simulink model "gm_parallel_prediction_and_cost_function_6phase"  (R2022a)
settings: Solver=FixedStepDiscrete  StartTime=0.0  StopTime=10.0  RelTol=1e-3
undefined symbols (not defined in the file or in its folder): f_c, L_d, L_q, L_x, L_y, p, psi_pm, R_ph
libraries: hdlmdlgenlib x2
(part 2 of 8)

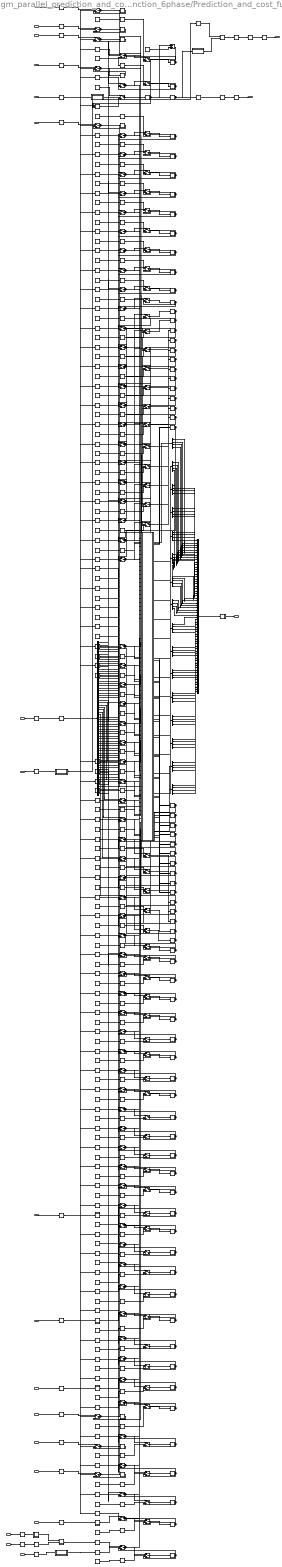
== system gm_parallel_prediction_and_cost_function_6phase/Prediction_and_cost_function ==
  Lq_AXI : Inport  OutDataTypeStr=single  PortDimensions=1  SampleTime=1e-08
  Ld_AXI : Inport  Port=2  OutDataTypeStr=single  PortDimensions=1  SampleTime=1e-08
  SampleTime_div_Ld_AXI : Inport  Port=3  OutDataTypeStr=single  PortDimensions=1  SampleTime=1e-08
  SampleTime_div_Lq_AXI : Inport  Port=4  OutDataTypeStr=single  PortDimensions=1  SampleTime=1e-08
  SampleTime_div_Lx_AXI : Inport  Port=5  OutDataTypeStr=single  PortDimensions=1  SampleTime=1e-08
  SampleTime_div_Ly_AXI : Inport  Port=6  OutDataTypeStr=single  PortDimensions=1  SampleTime=1e-08
  id_k_1 : Inport  Port=7  OutDataTypeStr=fixdt(1, 18, 11)  PortDimensions=1  SampleTime=1e-08
  iq_k_1 : Inport  Port=8  OutDataTypeStr=fixdt(1, 18, 11)  PortDimensions=1  SampleTime=1e-08
  ix_k_1 : Inport  Port=9  OutDataTypeStr=fixdt(1, 18, 11)  PortDimensions=1  SampleTime=1e-08
  iy_k_1 : Inport  Port=10  OutDataTypeStr=fixdt(1, 18, 11)  PortDimensions=1  SampleTime=1e-08
  Rs_AXI : Inport  Port=11  OutDataTypeStr=single  PortDimensions=1  SampleTime=1e-08
  omega_m_measured : Inport  Port=12  OutDataTypeStr=fixdt(1, 24, 11)  PortDimensions=1  SampleTime=1e-08
  pole_pairs_AXI : Inport  Port=13  OutDataTypeStr=single  PortDimensions=1  SampleTime=1e-08
  psiPM_AXI : Inport  Port=14  OutDataTypeStr=single  PortDimensions=1  SampleTime=1e-08
  valid_in : Inport  Port=15  OutDataTypeStr=boolean  PortDimensions=1  SampleTime=1e-08
  Reset : Inport  Port=16  OutDataTypeStr=boolean  PortDimensions=1  SampleTime=1e-08
  valid_in_ADC : Inport  Port=17  OutDataTypeStr=boolean  PortDimensions=1  SampleTime=1e-08
  dqxy_phase_voltage_per_switching_state : Inport  Port=18  OutDataTypeStr=fixdt(1, 24, 11)  PortDimensions=[64]  SampleTime=1e-08
  Compare To Constant : Subsystem  mask(Compare To Constant){relop=<=, const=double(4), OutDataTypeStr=boolean, ZeroCross=on}
      mask prompts: relop "Simulink:masks:Operator_MP"; const "Simulink:masks:ConstantValue_MP"; OutDataTypeStr "Simulink:masks:OutputDataType_MP"; ZeroCross "Simulink:masks:EnableZerocrossingDetection_MP"
      mask help: Simulink:masks:CompareToConstant_MD
      mask init:
      | OutDataTypeStr = 'boolean';
      | ZeroCross = 'on';
      | blkName = 'parallel_prediction_and_cost_function_6phase/Prediction_and_cost_function/Compare\nTo Constant';
      | const = double(4);
      | const_str = '4';
      | const_val = double(4);
      | relop = '<=';
      | setValue = 'boolean';
      | str = '<= 4';
      mask TypeOptions relop: == | ~= | < | <= | >= | >
      mask TypeOptions OutDataTypeStr: Simulink:masks:uint8 | Simulink:masks:boolean
      mask Callback ZeroCross: sl('zeroCrossEnable', gcbh);
      mask Display: disp(str)
  Data Type Conversion1 : Subsystem
      mask Display: disp('NFP\nconv');
  Data Type Conversion10 : Subsystem
      mask Display: disp('NFP\nconv');
  Data Type Conversion18 : Subsystem
      mask Display: disp('NFP\nconv');
  Data Type Conversion4 : Subsystem
      mask Display: disp('NFP\nconv');
  Data Type Conversion7 : Subsystem
      mask Display: disp('NFP\nconv');
  Data Type Conversion8 : Subsystem
      mask Display: disp('NFP\nconv');
  Data Type Conversion9 : Subsystem
      mask Display: disp('NFP\nconv');
  Delay{4..32,34..37,51,57,59..60,76..135} (97 alike) : Delay  DelayLength=double(1)  InitialCondition=0  SampleTime=1e-08
  Delay100_enbsw : Switch  Criteria=u2 ~= 0  Threshold=double(0)  OutDataTypeStr=single  SampleTime=1e-08  SaturateOnIntegerOverflow=off  InputSameDT=off
  Delay101_enbsw : Switch  Criteria=u2 ~= 0  Threshold=double(0)  OutDataTypeStr=single  SampleTime=1e-08  SaturateOnIntegerOverflow=off  InputSameDT=off
  Delay102_enbsw : Switch  Criteria=u2 ~= 0  Threshold=double(0)  OutDataTypeStr=single  SampleTime=1e-08  SaturateOnIntegerOverflow=off  InputSameDT=off
  Delay103_enbsw : Switch  Criteria=u2 ~= 0  Threshold=double(0)  OutDataTypeStr=single  SampleTime=1e-08  SaturateOnIntegerOverflow=off  InputSameDT=off
  Delay104_enbsw : Switch  Criteria=u2 ~= 0  Threshold=double(0)  OutDataTypeStr=single  SampleTime=1e-08  SaturateOnIntegerOverflow=off  InputSameDT=off
  Delay105_enbsw : Switch  Criteria=u2 ~= 0  Threshold=double(0)  OutDataTypeStr=single  SampleTime=1e-08  SaturateOnIntegerOverflow=off  InputSameDT=off
  Delay106_enbsw : Switch  Criteria=u2 ~= 0  Threshold=double(0)  OutDataTypeStr=single  SampleTime=1e-08  SaturateOnIntegerOverflow=off  InputSameDT=off
  Delay107_enbsw : Switch  Criteria=u2 ~= 0  Threshold=double(0)  OutDataTypeStr=single  SampleTime=1e-08  SaturateOnIntegerOverflow=off  InputSameDT=off
  Delay108_enbsw : Switch  Criteria=u2 ~= 0  Threshold=double(0)  OutDataTypeStr=single  SampleTime=1e-08  SaturateOnIntegerOverflow=off  InputSameDT=off
  Delay109_enbsw : Switch  Criteria=u2 ~= 0  Threshold=double(0)  OutDataTypeStr=single  SampleTime=1e-08  SaturateOnIntegerOverflow=off  InputSameDT=off
  Delay110_enbsw : Switch  Criteria=u2 ~= 0  Threshold=double(0)  OutDataTypeStr=single  SampleTime=1e-08  SaturateOnIntegerOverflow=off  InputSameDT=off
  Delay111_enbsw : Switch  Criteria=u2 ~= 0  Threshold=double(0)  OutDataTypeStr=single  SampleTime=1e-08  SaturateOnIntegerOverflow=off  InputSameDT=off
  Delay112_enbsw : Switch  Criteria=u2 ~= 0  Threshold=double(0)  OutDataTypeStr=single  SampleTime=1e-08  SaturateOnIntegerOverflow=off  InputSameDT=off
  Delay113_enbsw : Switch  Criteria=u2 ~= 0  Threshold=double(0)  OutDataTypeStr=single  SampleTime=1e-08  SaturateOnIntegerOverflow=off  InputSameDT=off
  Delay114_enbsw : Switch  Criteria=u2 ~= 0  Threshold=double(0)  OutDataTypeStr=single  SampleTime=1e-08  SaturateOnIntegerOverflow=off  InputSameDT=off
  Delay115_enbsw : Switch  Criteria=u2 ~= 0  Threshold=double(0)  OutDataTypeStr=single  SampleTime=1e-08  SaturateOnIntegerOverflow=off  InputSameDT=off
  Delay116_enbsw : Switch  Criteria=u2 ~= 0  Threshold=double(0)  OutDataTypeStr=single  SampleTime=1e-08  SaturateOnIntegerOverflow=off  InputSameDT=off
  Delay117_enbsw : Switch  Criteria=u2 ~= 0  Threshold=double(0)  OutDataTypeStr=single  SampleTime=1e-08  SaturateOnIntegerOverflow=off  InputSameDT=off
  Delay118_enbsw : Switch  Criteria=u2 ~= 0  Threshold=double(0)  OutDataTypeStr=single  SampleTime=1e-08  SaturateOnIntegerOverflow=off  InputSameDT=off
  Delay119_enbsw : Switch  Criteria=u2 ~= 0  Threshold=double(0)  OutDataTypeStr=single  SampleTime=1e-08  SaturateOnIntegerOverflow=off  InputSameDT=off
  Delay11_enbsw : Switch  Criteria=u2 ~= 0  Threshold=double(0)  OutDataTypeStr=single  SampleTime=1e-08  SaturateOnIntegerOverflow=off  InputSameDT=off
  Delay120_enbsw : Switch  Criteria=u2 ~= 0  Threshold=double(0)  OutDataTypeStr=single  SampleTime=1e-08  SaturateOnIntegerOverflow=off  InputSameDT=off
  Delay121_enbsw : Switch  Criteria=u2 ~= 0  Threshold=double(0)  OutDataTypeStr=single  SampleTime=1e-08  SaturateOnIntegerOverflow=off  InputSameDT=off
  Delay122_enbsw : Switch  Criteria=u2 ~= 0  Threshold=double(0)  OutDataTypeStr=single  SampleTime=1e-08  SaturateOnIntegerOverflow=off  InputSameDT=off
  Delay123_enbsw : Switch  Criteria=u2 ~= 0  Threshold=double(0)  OutDataTypeStr=single  SampleTime=1e-08  SaturateOnIntegerOverflow=off  InputSameDT=off
  Delay124_enbsw : Switch  Criteria=u2 ~= 0  Threshold=double(0)  OutDataTypeStr=single  SampleTime=1e-08  SaturateOnIntegerOverflow=off  InputSameDT=off
  Delay125_enbsw : Switch  Criteria=u2 ~= 0  Threshold=double(0)  OutDataTypeStr=single  SampleTime=1e-08  SaturateOnIntegerOverflow=off  InputSameDT=off
  Delay126_enbsw : Switch  Criteria=u2 ~= 0  Threshold=double(0)  OutDataTypeStr=single  SampleTime=1e-08  SaturateOnIntegerOverflow=off  InputSameDT=off
  Delay127_enbsw : Switch  Criteria=u2 ~= 0  Threshold=double(0)  OutDataTypeStr=single  SampleTime=1e-08  SaturateOnIntegerOverflow=off  InputSameDT=off
  Delay128_enbsw : Switch  Criteria=u2 ~= 0  Threshold=double(0)  OutDataTypeStr=single  SampleTime=1e-08  SaturateOnIntegerOverflow=off  InputSameDT=off
  Delay129_enbsw : Switch  Criteria=u2 ~= 0  Threshold=double(0)  OutDataTypeStr=single  SampleTime=1e-08  SaturateOnIntegerOverflow=off  InputSameDT=off
  Delay130_enbsw : Switch  Criteria=u2 ~= 0  Threshold=double(0)  OutDataTypeStr=single  SampleTime=1e-08  SaturateOnIntegerOverflow=off  InputSameDT=off
  Delay131_enbsw : Switch  Criteria=u2 ~= 0  Threshold=double(0)  OutDataTypeStr=single  SampleTime=1e-08  SaturateOnIntegerOverflow=off  InputSameDT=off
  Delay132_enbsw : Switch  Criteria=u2 ~= 0  Threshold=double(0)  OutDataTypeStr=single  SampleTime=1e-08  SaturateOnIntegerOverflow=off  InputSameDT=off
  Delay133_enbsw : Switch  Criteria=u2 ~= 0  Threshold=double(0)  OutDataTypeStr=single  SampleTime=1e-08  SaturateOnIntegerOverflow=off  InputSameDT=off
  Delay134_enbsw : Switch  Criteria=u2 ~= 0  Threshold=double(0)  OutDataTypeStr=single  SampleTime=1e-08  SaturateOnIntegerOverflow=off  InputSameDT=off
  Delay135_enbsw : Switch  Criteria=u2 ~= 0  Threshold=double(0)  OutDataTypeStr=single  SampleTime=1e-08  SaturateOnIntegerOverflow=off  InputSameDT=off
  Delay13_enbsw : Switch  Criteria=u2 ~= 0  Threshold=double(0)  OutDataTypeStr=single  SampleTime=1e-08  SaturateOnIntegerOverflow=off  InputSameDT=off
  Delay14_enbsw : Switch  Criteria=u2 ~= 0  Threshold=double(0)  OutDataTypeStr=single  SampleTime=1e-08  SaturateOnIntegerOverflow=off  InputSameDT=off
  Delay15_enbsw : Switch  Criteria=u2 ~= 0  Threshold=double(0)  OutDataTypeStr=single  SampleTime=1e-08  SaturateOnIntegerOverflow=off  InputSameDT=off
  Delay16_enbsw : Switch  Criteria=u2 ~= 0  Threshold=double(0)  OutDataTypeStr=single  SampleTime=1e-08  SaturateOnIntegerOverflow=off  InputSameDT=off
  Delay4_enbsw : Switch  Criteria=u2 ~= 0  Threshold=double(0)  OutDataTypeStr=single  SampleTime=1e-08  SaturateOnIntegerOverflow=off  InputSameDT=off
  Delay58 : Delay  DelayLength=double(3)  InitialCondition=0  SampleTime=1e-08
  Delay5_enbsw : Switch  Criteria=u2 ~= 0  Threshold=double(0)  OutDataTypeStr=single  SampleTime=1e-08  SaturateOnIntegerOverflow=off  InputSameDT=off
  Delay6_enbsw : Switch  Criteria=u2 ~= 0  Threshold=double(0)  OutDataTypeStr=single  SampleTime=1e-08  SaturateOnIntegerOverflow=off  InputSameDT=off
  Delay76_enbsw : Switch  Criteria=u2 ~= 0  Threshold=double(0)  OutDataTypeStr=single  SampleTime=1e-08  SaturateOnIntegerOverflow=off  InputSameDT=off
  Delay77_enbsw : Switch  Criteria=u2 ~= 0  Threshold=double(0)  OutDataTypeStr=single  SampleTime=1e-08  SaturateOnIntegerOverflow=off  InputSameDT=off
  Delay78_enbsw : Switch  Criteria=u2 ~= 0  Threshold=double(0)  OutDataTypeStr=single  SampleTime=1e-08  SaturateOnIntegerOverflow=off  InputSameDT=off
  Delay79_enbsw : Switch  Criteria=u2 ~= 0  Threshold=double(0)  OutDataTypeStr=single  SampleTime=1e-08  SaturateOnIntegerOverflow=off  InputSameDT=off
  Delay7_enbsw : Switch  Criteria=u2 ~= 0  Threshold=double(0)  OutDataTypeStr=single  SampleTime=1e-08  SaturateOnIntegerOverflow=off  InputSameDT=off
  Delay80_enbsw : Switch  Criteria=u2 ~= 0  Threshold=double(0)  OutDataTypeStr=single  SampleTime=1e-08  SaturateOnIntegerOverflow=off  InputSameDT=off
  Delay81_enbsw : Switch  Criteria=u2 ~= 0  Threshold=double(0)  OutDataTypeStr=single  SampleTime=1e-08  SaturateOnIntegerOverflow=off  InputSameDT=off
  Delay82_enbsw : Switch  Criteria=u2 ~= 0  Threshold=double(0)  OutDataTypeStr=single  SampleTime=1e-08  SaturateOnIntegerOverflow=off  InputSameDT=off
  Delay83_enbsw : Switch  Criteria=u2 ~= 0  Threshold=double(0)  OutDataTypeStr=single  SampleTime=1e-08  SaturateOnIntegerOverflow=off  InputSameDT=off
  Delay84_enbsw : Switch  Criteria=u2 ~= 0  Threshold=double(0)  OutDataTypeStr=single  SampleTime=1e-08  SaturateOnIntegerOverflow=off  InputSameDT=off
  Delay85_enbsw : Switch  Criteria=u2 ~= 0  Threshold=double(0)  OutDataTypeStr=single  SampleTime=1e-08  SaturateOnIntegerOverflow=off  InputSameDT=off
  Delay86_enbsw : Switch  Criteria=u2 ~= 0  Threshold=double(0)  OutDataTypeStr=single  SampleTime=1e-08  SaturateOnIntegerOverflow=off  InputSameDT=off
  Delay87_enbsw : Switch  Criteria=u2 ~= 0  Threshold=double(0)  OutDataTypeStr=single  SampleTime=1e-08  SaturateOnIntegerOverflow=off  InputSameDT=off
  Delay88_enbsw : Switch  Criteria=u2 ~= 0  Threshold=double(0)  OutDataTypeStr=single  SampleTime=1e-08  SaturateOnIntegerOverflow=off  InputSameDT=off
  Delay89_enbsw : Switch  Criteria=u2 ~= 0  Threshold=double(0)  OutDataTypeStr=single  SampleTime=1e-08  SaturateOnIntegerOverflow=off  InputSameDT=off
  Delay90_enbsw : Switch  Criteria=u2 ~= 0  Threshold=double(0)  OutDataTypeStr=single  SampleTime=1e-08  SaturateOnIntegerOverflow=off  InputSameDT=off
  Delay91_enbsw : Switch  Criteria=u2 ~= 0  Threshold=double(0)  OutDataTypeStr=single  SampleTime=1e-08  SaturateOnIntegerOverflow=off  InputSameDT=off
  Delay92_enbsw : Switch  Criteria=u2 ~= 0  Threshold=double(0)  OutDataTypeStr=single  SampleTime=1e-08  SaturateOnIntegerOverflow=off  InputSameDT=off
  Delay93_enbsw : Switch  Criteria=u2 ~= 0  Threshold=double(0)  OutDataTypeStr=single  SampleTime=1e-08  SaturateOnIntegerOverflow=off  InputSameDT=off
  Delay94_enbsw : Switch  Criteria=u2 ~= 0  Threshold=double(0)  OutDataTypeStr=single  SampleTime=1e-08  SaturateOnIntegerOverflow=off  InputSameDT=off
  Delay95_enbsw : Switch  Criteria=u2 ~= 0  Threshold=double(0)  OutDataTypeStr=single  SampleTime=1e-08  SaturateOnIntegerOverflow=off  InputSameDT=off
  Delay96_enbsw : Switch  Criteria=u2 ~= 0  Threshold=double(0)  OutDataTypeStr=single  SampleTime=1e-08  SaturateOnIntegerOverflow=off  InputSameDT=off
  Delay97_enbsw : Switch  Criteria=u2 ~= 0  Threshold=double(0)  OutDataTypeStr=single  SampleTime=1e-08  SaturateOnIntegerOverflow=off  InputSameDT=off
  Delay98_enbsw : Switch  Criteria=u2 ~= 0  Threshold=double(0)  OutDataTypeStr=single  SampleTime=1e-08  SaturateOnIntegerOverflow=off  InputSameDT=off
  Delay99_enbsw : Switch  Criteria=u2 ~= 0  Threshold=double(0)  OutDataTypeStr=single  SampleTime=1e-08  SaturateOnIntegerOverflow=off  InputSameDT=off
  Detect Rise Positive : Subsystem  mask(Detect Rise Positive){vinit=double(0), InputProcessing=Elements as channels (sample based), OutDataTypeStr=boolean}
      mask prompts: vinit "Simulink:masks:InitialCondition_MP"; InputProcessing "Simulink:masks:InputProcessing_MP"; OutDataTypeStr "Simulink:masks:OutputDataType_MP"
      mask help: Simulink:masks:DetectRisePositive_MD
      mask init:
      | InputProcessing = 'Elements as channels (sample based)';
      | OutDataTypeStr = 'boolean';
      | vinit = double(0);
      mask TypeOptions InputProcessing: Simulink:masks:ColumnsAsChannelsFrameBased | Simulink:masks:ElementsAsChannelsSampleBased
      mask TypeOptions OutDataTypeStr: Simulink:masks:uint8 | Simulink:masks:boolean
      mask Display: fprintf('U > 0\n&  NOT\nU/z > 0')
  Detect Rise Positive1 : Subsystem  mask(Detect Rise Positive){vinit=double(0), InputProcessing=Elements as channels (sample based), OutDataTypeStr=boolean}
      mask prompts: vinit "Simulink:masks:InitialCondition_MP"; InputProcessing "Simulink:masks:InputProcessing_MP"; OutDataTypeStr "Simulink:masks:OutputDataType_MP"
      mask help: Simulink:masks:DetectRisePositive_MD
      mask init:
      | InputProcessing = 'Elements as channels (sample based)';
      | OutDataTypeStr = 'boolean';
      | vinit = double(0);
      mask TypeOptions InputProcessing: Simulink:masks:ColumnsAsChannelsFrameBased | Simulink:masks:ElementsAsChannelsSampleBased
      mask TypeOptions OutDataTypeStr: Simulink:masks:uint8 | Simulink:masks:boolean
      mask Display: fprintf('U > 0\n&  NOT\nU/z > 0')
  Detect Rise Positive2 : Subsystem  mask(Detect Rise Positive){vinit=double(0), InputProcessing=Elements as channels (sample based), OutDataTypeStr=boolean}
      mask prompts: vinit "Simulink:masks:InitialCondition_MP"; InputProcessing "Simulink:masks:InputProcessing_MP"; OutDataTypeStr "Simulink:masks:OutputDataType_MP"
      mask help: Simulink:masks:DetectRisePositive_MD
      mask init:
      | InputProcessing = 'Elements as channels (sample based)';
      | OutDataTypeStr = 'boolean';
      | vinit = double(0);
      mask TypeOptions InputProcessing: Simulink:masks:ColumnsAsChannelsFrameBased | Simulink:masks:ElementsAsChannelsSampleBased
      mask TypeOptions OutDataTypeStr: Simulink:masks:uint8 | Simulink:masks:boolean
      mask Display: fprintf('U > 0\n&  NOT\nU/z > 0')
  HDL Counter : Delay  DelayLength=double(1)  InitialCondition=0  SampleTime=1e-08
  HDL Counter_out1 : hdlmdlgenlib/Buffer
      settings: SourceProductBaseCode=SL
  Logical Operator : Logic  AllPortsSameDT=off  OutDataTypeStr=boolean  SampleTime=1e-08
  Product : Subsystem
      mask Display: disp('NFP\nmul');
  Product_outbuff : hdlmdlgenlib/Buffer
      settings: SourceProductBaseCode=SL
  Subsystem : Subsystem
  Switch_on{4..13,15..21,31..90} (77 alike) : Switch  Threshold=double(1)  OutDataTypeStr=single  RndMeth=Simplest  SampleTime=1e-08  SaturateOnIntegerOverflow=off  InputSameDT=off
  adder : Sum  AccumDataTypeStr=int32  OutDataTypeStr=int32  SampleTime=1e-08
  const : Constant  Value=0  VectorParams1D=off  OutDataTypeStr=int32  SampleTime=1e-08
  delayMatch : Delay  DelayLength=double(36)  InitialCondition=0  SampleTime=1e-08
  delayMatch1 : Delay  DelayLength=double(36)  InitialCondition=0  SampleTime=1e-08
  delayMatch{2..130,133..140} (137 alike) : Delay  DelayLength=double(6)  InitialCondition=0  SampleTime=1e-08
  delayMatch131 : Delay  DelayLength=double(12)  InitialCondition=0  SampleTime=1e-08
  delayMatch132 : Delay  DelayLength=double(12)  InitialCondition=0  SampleTime=1e-08
  delayMatch141 : Delay  DelayLength=double(11)  InitialCondition=0  SampleTime=1e-08
  delayMatch142 : Delay  DelayLength=double(11)  InitialCondition=0  SampleTime=1e-08
  mux : Mux  Inputs=64
  stateControl{,1..68} (69 alike) : Constant  OutDataTypeStr=boolean  SampleTime=1e-08
  step_value : Constant  VectorParams1D=off  OutDataTypeStr=int32  SampleTime=1e-08
  switchEnable : MultiPortSwitch  DataPortOrder=Zero-based contiguous  Inputs=2  DiagnosticForDefault=None  zeroidx=on  OutDataTypeStr=int32  SampleTime=1e-08  SaturateOnIntegerOverflow=off  InputSameDT=off
  switchReset : Switch  Criteria=u2 ~= 0  Threshold=double(0)  OutDataTypeStr=int32  SampleTime=1e-08  SaturateOnIntegerOverflow=off  InputSameDT=off
  t : Demux  Outputs=64
  t{1..16} (16 alike) : Demux
  done : Outport  SampleTime=1e-08
  Index : Outport  Port=2  SampleTime=1e-08
  Prediction : Outport  Port=3  SampleTime=1e-08
  wires:
  Lq_AXI/1 -> Delay34/1
  Ld_AXI/1 -> Delay36/1
  SampleTime_div_Ld_AXI/1 -> Delay23/1
  SampleTime_div_Lq_AXI/1 -> Delay24/1
  SampleTime_div_Lx_AXI/1 -> Delay25/1
  SampleTime_div_Ly_AXI/1 -> Delay26/1
  id_k_1/1 -> Delay27/1
  iq_k_1/1 -> Delay28/1
  ix_k_1/1 -> Delay29/1
  iy_k_1/1 -> Delay30/1
  Rs_AXI/1 -> Delay31/1
  omega_m_measured/1 -> Delay51/1
  pole_pairs_AXI/1 -> Delay35/1
  psiPM_AXI/1 -> Delay37/1
  valid_in/1 -> Delay21/1
  Reset/1 -> Delay57/1
  valid_in_ADC/1 -> Delay60/1
  dqxy_phase_voltage_per_switching_state/1 -> Delay32/1
  Compare To Constant/1(y) -> Logical Operator/2
  Delay21/1 -> Detect Rise Positive/1(U)
  Delay22/1 -> Logical Operator/1
  Delay23/1 -> Switch_on21/1
  Delay24/1 -> Switch_on20/1
  Delay25/1 -> Switch_on19/1
  Delay26/1 -> Switch_on18/1
  Delay27/1 -> Data Type Conversion7/1(In1)
  Delay28/1 -> Data Type Conversion8/1(In1)
  Delay29/1 -> Data Type Conversion9/1(In1)
  Delay30/1 -> Data Type Conversion10/1(In1)
  Delay31/1 -> Switch_on12/1
  Delay32/1 -> Data Type Conversion1/1(In1)
  Delay34/1 -> Switch_on10/1
  delayMatch130/1 -> Product/2(In2)
  Delay36/1 -> Switch_on9/1
  Delay37/1 -> Switch_on8/1
  Delay51/1 -> Data Type Conversion4/1(In1)
  Delay57/1 -> Detect Rise Positive1/1(U)
  delayMatch141/1 -> done/1
  delayMatch142/1 -> Index/1
  Delay60/1 -> Detect Rise Positive2/1(U)
  delayMatch3/1 -> Switch_on90/2
  Detect Rise Positive1/1(Y) -> switchReset/2
  delayMatch132/1 -> Switch_on11/2
  HDL Counter_out1/1 -> Delay59/1, Compare To Constant/1(u)
  Logical Operator/1 -> Delay58/1
  mux/1 -> Data Type Conversion18/1(In1)
  Product_outbuff/1 -> Switch_on11/1
  Subsystem/1(Prediction_1) -> t1/1
  Subsystem/2(Prediction_2) -> t2/1
  Subsystem/3(Prediction_3) -> t3/1
  Subsystem/4(Prediction_4) -> t4/1
  Subsystem/5(Prediction_5) -> t5/1
  Subsystem/6(Prediction_6) -> t6/1
  Subsystem/7(Prediction_7) -> t7/1
  Subsystem/8(Prediction_8) -> t8/1
  Subsystem/9(Prediction_9) -> t9/1
  Subsystem/10(Prediction_10) -> t10/1
  Subsystem/11(Prediction_11) -> t11/1
  Subsystem/12(Prediction_12) -> t12/1
  Subsystem/13(Prediction_13) -> t13/1
  Subsystem/14(Prediction_14) -> t14/1
  Subsystem/15(Prediction_15) -> t15/1
  Subsystem/16(Prediction_16) -> t16/1
  Switch_on10/1 -> Subsystem/71(Lq15), Delay10/1
  Switch_on12/1 -> Subsystem/69(Rs15), Delay12/1
  Switch_on18/1 -> Subsystem/64(SampleTime_div_Ly15), Delay17/1
  Switch_on19/1 -> Subsystem/63(SampleTime_div_Lx15), Delay18/1
  Switch_on20/1 -> Subsystem/62(SampleTime_div_Lq15), Delay19/1
  Switch_on21/1 -> Subsystem/61(SampleTime_div_Ld15), Delay20/1
  Switch_on8/1 -> Subsystem/73(psiPM15), Delay8/1
  Switch_on9/1 -> Subsystem/72(Ld15), Delay9/1
  HDL Counter/1 -> HDL Counter_out1/1, switchEnable/2, adder/1
  const/1 -> switchReset/1
  step_value/1 -> adder/2
  t/1 -> Switch_on90/1
  t/2 -> Switch_on89/1
  t/3 -> Switch_on88/1
  t/4 -> Switch_on87/1
  t/5 -> Switch_on86/1
  t/6 -> Switch_on85/1
  t/7 -> Switch_on84/1
  t/8 -> Switch_on83/1
  t/9 -> Switch_on82/1
  t/10 -> Switch_on81/1
  t/11 -> Switch_on80/1
  t/12 -> Switch_on79/1
  t/13 -> Switch_on78/1
  t/14 -> Switch_on77/1
  t/15 -> Switch_on76/1
  t/16 -> Switch_on75/1
  t/17 -> Switch_on74/1
  t/18 -> Switch_on73/1
  t/19 -> Switch_on72/1
  t/20 -> Switch_on71/1
  t/21 -> Switch_on70/1
  t/22 -> Switch_on69/1
  t/23 -> Switch_on68/1
  t/24 -> Switch_on67/1
  t/25 -> Switch_on66/1
  t/26 -> Switch_on65/1
  t/27 -> Switch_on64/1
  t/28 -> Switch_on63/1
  t/29 -> Switch_on62/1
  t/30 -> Switch_on61/1
  t/31 -> Switch_on60/1
  t/32 -> Switch_on59/1
  t/33 -> Switch_on58/1
  t/34 -> Switch_on57/1
  t/35 -> Switch_on56/1
  t/36 -> Switch_on55/1
  t/37 -> Switch_on54/1
  t/38 -> Switch_on53/1
  t/39 -> Switch_on52/1
  t/40 -> Switch_on51/1
  t/41 -> Switch_on50/1
  t/42 -> Switch_on49/1
  t/43 -> Switch_on48/1
  t/44 -> Switch_on47/1
  t/45 -> Switch_on46/1
  t/46 -> Switch_on45/1
  t/47 -> Switch_on44/1
  t/48 -> Switch_on43/1
  t/49 -> Switch_on42/1
  t/50 -> Switch_on41/1
  t/51 -> Switch_on40/1
  t/52 -> Switch_on39/1
  t/53 -> Switch_on38/1
  t/54 -> Switch_on37/1
  t/55 -> Switch_on36/1
  t/56 -> Switch_on35/1
  t/57 -> Switch_on34/1
  t/58 -> Switch_on33/1
  t/59 -> Switch_on32/1
  t/60 -> Switch_on31/1
  t/61 -> Switch_on7/1
  t/62 -> Switch_on6/1
  t/63 -> Switch_on5/1
  t/64 -> Switch_on4/1
  t1/1 -> mux/1
  t1/2 -> mux/2
  t1/3 -> mux/3
  t1/4 -> mux/4
  t2/1 -> mux/5
  t2/2 -> mux/6
  t2/3 -> mux/7
  t2/4 -> mux/8
  t3/1 -> mux/9
  t3/2 -> mux/10
  t3/3 -> mux/11
  t3/4 -> mux/12
  t4/1 -> mux/13
  t4/2 -> mux/14
  t4/3 -> mux/15
  t4/4 -> mux/16
  t5/1 -> mux/17
  t5/2 -> mux/18
  t5/3 -> mux/19
  t5/4 -> mux/20
  t6/1 -> mux/21
  t6/2 -> mux/22
  t6/3 -> mux/23
  t6/4 -> mux/24
  t7/1 -> mux/25
  t7/2 -> mux/26
  t7/3 -> mux/27
  t7/4 -> mux/28
  t8/1 -> mux/29
  t8/2 -> mux/30
  t8/3 -> mux/31
  t8/4 -> mux/32
  t9/1 -> mux/33
  t9/2 -> mux/34
  t9/3 -> mux/35
  t9/4 -> mux/36
  t10/1 -> mux/37
  t10/2 -> mux/38
  t10/3 -> mux/39
  t10/4 -> mux/40
  t11/1 -> mux/41
  t11/2 -> mux/42
  t11/3 -> mux/43
  t11/4 -> mux/44
  t12/1 -> mux/45
  t12/2 -> mux/46
  t12/3 -> mux/47
  t12/4 -> mux/48
  t13/1 -> mux/49
  t13/2 -> mux/50
  t13/3 -> mux/51
  t13/4 -> mux/52
  t14/1 -> mux/53
  t14/2 -> mux/54
  t14/3 -> mux/55
  t14/4 -> mux/56
  t15/1 -> mux/57
  t15/2 -> mux/58
  t15/3 -> mux/59
  t15/4 -> mux/60
  t16/1 -> mux/61
  t16/2 -> mux/62
  t16/3 -> mux/63
  t16/4 -> mux/64
  Delay58/1 -> delayMatch/1
  Delay59/1 -> delayMatch1/1
  Data Type Conversion1/1(Out1) -> t/1
  Data Type Conversion10/1(Out1) -> Switch_on13/1
  Data Type Conversion18/1(Out1) -> Prediction/1
  Data Type Conversion4/1(Out1) -> Product/1(In1)
  Data Type Conversion7/1(Out1) -> Switch_on17/1
  Data Type Conversion8/1(Out1) -> Switch_on16/1
  Data Type Conversion9/1(Out1) -> Switch_on15/1
  Product/1(Out1) -> Product_outbuff/1
  delayMatch2/1 -> Delay135_enbsw/2
  delayMatch4/1 -> Delay134_enbsw/2
  delayMatch6/1 -> Delay133_enbsw/2
  delayMatch8/1 -> Delay132_enbsw/2
  delayMatch10/1 -> Delay131_enbsw/2
  delayMatch12/1 -> Delay130_enbsw/2
  delayMatch14/1 -> Delay129_enbsw/2
  delayMatch16/1 -> Delay128_enbsw/2
  delayMatch18/1 -> Delay127_enbsw/2
  delayMatch20/1 -> Delay126_enbsw/2
  delayMatch22/1 -> Delay125_enbsw/2
  delayMatch24/1 -> Delay124_enbsw/2
  delayMatch26/1 -> Delay123_enbsw/2
  delayMatch28/1 -> Delay122_enbsw/2
  delayMatch30/1 -> Delay121_enbsw/2
  delayMatch32/1 -> Delay120_enbsw/2
  delayMatch34/1 -> Delay119_enbsw/2
  delayMatch36/1 -> Delay118_enbsw/2
  delayMatch38/1 -> Delay117_enbsw/2
  delayMatch40/1 -> Delay116_enbsw/2
  delayMatch42/1 -> Delay115_enbsw/2
  delayMatch44/1 -> Delay114_enbsw/2
  delayMatch46/1 -> Delay113_enbsw/2
  delayMatch48/1 -> Delay112_enbsw/2
  delayMatch50/1 -> Delay111_enbsw/2
  delayMatch52/1 -> Delay110_enbsw/2
  delayMatch54/1 -> Delay109_enbsw/2
  delayMatch56/1 -> Delay108_enbsw/2
  delayMatch58/1 -> Delay107_enbsw/2
  delayMatch60/1 -> Delay106_enbsw/2
  delayMatch62/1 -> Delay105_enbsw/2
  delayMatch64/1 -> Delay104_enbsw/2
  delayMatch66/1 -> Delay103_enbsw/2
  delayMatch68/1 -> Delay102_enbsw/2
  delayMatch70/1 -> Delay101_enbsw/2
  delayMatch72/1 -> Delay100_enbsw/2
  delayMatch74/1 -> Delay99_enbsw/2
  delayMatch76/1 -> Delay98_enbsw/2
  delayMatch78/1 -> Delay97_enbsw/2
  delayMatch80/1 -> Delay96_enbsw/2
  delayMatch82/1 -> Delay95_enbsw/2
  delayMatch84/1 -> Delay94_enbsw/2
  delayMatch86/1 -> Delay93_enbsw/2
  delayMatch88/1 -> Delay92_enbsw/2
  delayMatch90/1 -> Delay91_enbsw/2
  delayMatch92/1 -> Delay90_enbsw/2
  delayMatch94/1 -> Delay89_enbsw/2
  delayMatch96/1 -> Delay88_enbsw/2
  delayMatch98/1 -> Delay87_enbsw/2
  delayMatch100/1 -> Delay86_enbsw/2
  delayMatch102/1 -> Delay85_enbsw/2
  delayMatch104/1 -> Delay84_enbsw/2
  delayMatch106/1 -> Delay83_enbsw/2
  delayMatch108/1 -> Delay82_enbsw/2
  delayMatch110/1 -> Delay81_enbsw/2
  delayMatch112/1 -> Delay80_enbsw/2
  delayMatch114/1 -> Delay79_enbsw/2
  delayMatch116/1 -> Delay78_enbsw/2
  delayMatch118/1 -> Delay77_enbsw/2
  delayMatch120/1 -> Delay76_enbsw/2
  delayMatch122/1 -> Delay16_enbsw/2
  delayMatch124/1 -> Delay15_enbsw/2
  delayMatch126/1 -> Delay14_enbsw/2
  delayMatch128/1 -> Delay13_enbsw/2
  delayMatch131/1 -> Delay11_enbsw/2
  delayMatch133/1 -> Delay7_enbsw/2
  delayMatch135/1 -> Delay6_enbsw/2
  delayMatch137/1 -> Delay5_enbsw/2
  delayMatch139/1 -> Delay4_enbsw/2
  stateControl/1 -> delayMatch2/1
  delayMatch5/1 -> Switch_on89/2
  stateControl1/1 -> delayMatch4/1
  delayMatch7/1 -> Switch_on88/2
  stateControl2/1 -> delayMatch6/1
  delayMatch9/1 -> Switch_on87/2
  stateControl3/1 -> delayMatch8/1
  delayMatch11/1 -> Switch_on86/2
  stateControl4/1 -> delayMatch10/1
  delayMatch13/1 -> Switch_on85/2
  stateControl5/1 -> delayMatch12/1
  delayMatch15/1 -> Switch_on84/2
  stateControl6/1 -> delayMatch14/1
  delayMatch17/1 -> Switch_on83/2
  stateControl7/1 -> delayMatch16/1
  delayMatch19/1 -> Switch_on82/2
  stateControl8/1 -> delayMatch18/1
  delayMatch21/1 -> Switch_on81/2
  stateControl9/1 -> delayMatch20/1
  delayMatch23/1 -> Switch_on80/2
  stateControl10/1 -> delayMatch22/1
  delayMatch25/1 -> Switch_on79/2
  stateControl11/1 -> delayMatch24/1
  delayMatch27/1 -> Switch_on78/2
  stateControl12/1 -> delayMatch26/1
  delayMatch29/1 -> Switch_on77/2
  stateControl13/1 -> delayMatch28/1
  delayMatch31/1 -> Switch_on76/2
  stateControl14/1 -> delayMatch30/1
  delayMatch33/1 -> Switch_on75/2
  stateControl15/1 -> delayMatch32/1
  delayMatch35/1 -> Switch_on74/2
  stateControl16/1 -> delayMatch34/1
  delayMatch37/1 -> Switch_on73/2
  stateControl17/1 -> delayMatch36/1
  delayMatch39/1 -> Switch_on72/2
  stateControl18/1 -> delayMatch38/1
  delayMatch41/1 -> Switch_on71/2
  stateControl19/1 -> delayMatch40/1
  delayMatch43/1 -> Switch_on70/2
  stateControl20/1 -> delayMatch42/1
  delayMatch45/1 -> Switch_on69/2
  stateControl21/1 -> delayMatch44/1
  delayMatch47/1 -> Switch_on68/2
  stateControl22/1 -> delayMatch46/1
  delayMatch49/1 -> Switch_on67/2
  stateControl23/1 -> delayMatch48/1
  delayMatch51/1 -> Switch_on66/2
  stateControl24/1 -> delayMatch50/1
  delayMatch53/1 -> Switch_on65/2
  stateControl25/1 -> delayMatch52/1
  delayMatch55/1 -> Switch_on64/2
  stateControl26/1 -> delayMatch54/1
  delayMatch57/1 -> Switch_on63/2
  stateControl27/1 -> delayMatch56/1
  delayMatch59/1 -> Switch_on62/2
  stateControl28/1 -> delayMatch58/1
  delayMatch61/1 -> Switch_on61/2
  stateControl29/1 -> delayMatch60/1
  delayMatch63/1 -> Switch_on60/2
  stateControl30/1 -> delayMatch62/1
  delayMatch65/1 -> Switch_on59/2
  stateControl31/1 -> delayMatch64/1
  delayMatch67/1 -> Switch_on58/2
  stateControl32/1 -> delayMatch66/1
  delayMatch69/1 -> Switch_on57/2
  stateControl33/1 -> delayMatch68/1
  delayMatch71/1 -> Switch_on56/2
  stateControl34/1 -> delayMatch70/1
  delayMatch73/1 -> Switch_on55/2
  stateControl35/1 -> delayMatch72/1
  delayMatch75/1 -> Switch_on54/2
  stateControl36/1 -> delayMatch74/1
  delayMatch77/1 -> Switch_on53/2
  stateControl37/1 -> delayMatch76/1
  delayMatch79/1 -> Switch_on52/2
  stateControl38/1 -> delayMatch78/1
  delayMatch81/1 -> Switch_on51/2
  stateControl39/1 -> delayMatch80/1
  delayMatch83/1 -> Switch_on50/2
  stateControl40/1 -> delayMatch82/1
  delayMatch85/1 -> Switch_on49/2
  stateControl41/1 -> delayMatch84/1
  delayMatch87/1 -> Switch_on48/2
  stateControl42/1 -> delayMatch86/1
  delayMatch89/1 -> Switch_on47/2
  stateControl43/1 -> delayMatch88/1
  delayMatch91/1 -> Switch_on46/2
  stateControl44/1 -> delayMatch90/1
  delayMatch93/1 -> Switch_on45/2
  stateControl45/1 -> delayMatch92/1
  delayMatch95/1 -> Switch_on44/2
  stateControl46/1 -> delayMatch94/1
  delayMatch97/1 -> Switch_on43/2
  stateControl47/1 -> delayMatch96/1
  delayMatch99/1 -> Switch_on42/2
  stateControl48/1 -> delayMatch98/1
  delayMatch101/1 -> Switch_on41/2
  stateControl49/1 -> delayMatch100/1
  delayMatch103/1 -> Switch_on40/2
  stateControl50/1 -> delayMatch102/1
  delayMatch105/1 -> Switch_on39/2
  stateControl51/1 -> delayMatch104/1
  delayMatch107/1 -> Switch_on38/2
  stateControl52/1 -> delayMatch106/1
  delayMatch109/1 -> Switch_on37/2
  stateControl53/1 -> delayMatch108/1
  delayMatch111/1 -> Switch_on36/2
  stateControl54/1 -> delayMatch110/1
  delayMatch113/1 -> Switch_on35/2
  stateControl55/1 -> delayMatch112/1
  delayMatch115/1 -> Switch_on34/2
  stateControl56/1 -> delayMatch114/1
  delayMatch117/1 -> Switch_on33/2
  stateControl57/1 -> delayMatch116/1
  delayMatch119/1 -> Switch_on32/2
  stateControl58/1 -> delayMatch118/1
  delayMatch121/1 -> Switch_on31/2
  stateControl59/1 -> delayMatch120/1
  delayMatch123/1 -> Switch_on17/2
  stateControl60/1 -> delayMatch122/1
  delayMatch125/1 -> Switch_on16/2
  stateControl61/1 -> delayMatch124/1
  delayMatch127/1 -> Switch_on15/2
  stateControl62/1 -> delayMatch126/1
  delayMatch129/1 -> Switch_on13/2
  stateControl63/1 -> delayMatch128/1
  delayMatch134/1 -> Switch_on7/2
  Delay35/1 -> delayMatch130/1
  stateControl64/1 -> delayMatch131/1
  Detect Rise Positive2/1(Y) -> delayMatch132/1
  stateControl65/1 -> delayMatch133/1
  delayMatch136/1 -> Switch_on6/2
  stateControl66/1 -> delayMatch135/1
  delayMatch138/1 -> Switch_on5/2
  stateControl67/1 -> delayMatch137/1
  delayMatch140/1 -> Switch_on4/2
  stateControl68/1 -> delayMatch139/1
  Detect Rise Positive/1(Y) -> delayMatch140/1, delayMatch138/1, delayMatch136/1, delayMatch134/1, delayMatch129/1, delayMatch127/1, delayMatch125/1, delayMatch123/1, delayMatch121/1, delayMatch119/1, delayMatch117/1, delayMatch115/1, delayMatch113/1, delayMatch111/1, delayMatch109/1, delayMatch107/1, delayMatch105/1, delayMatch103/1, delayMatch101/1, delayMatch99/1, delayMatch97/1, delayMatch95/1, delayMatch93/1, delayMatch91/1, delayMatch89/1, delayMatch87/1, delayMatch85/1, delayMatch83/1, delayMatch81/1, delayMatch79/1, delayMatch77/1, delayMatch75/1, delayMatch73/1, delayMatch71/1, delayMatch69/1, delayMatch67/1, delayMatch65/1, delayMatch63/1, delayMatch61/1, delayMatch59/1, delayMatch57/1, delayMatch55/1, delayMatch53/1, delayMatch51/1, delayMatch49/1, delayMatch47/1, delayMatch45/1, delayMatch43/1, delayMatch41/1, delayMatch39/1, delayMatch37/1, delayMatch35/1, delayMatch33/1, delayMatch31/1, delayMatch29/1, delayMatch27/1, delayMatch25/1, delayMatch23/1, delayMatch21/1, delayMatch19/1, delayMatch17/1, delayMatch15/1, delayMatch13/1, delayMatch11/1, delayMatch9/1, delayMatch7/1, delayMatch5/1, delayMatch3/1, Delay22/1, switchEnable/1, Switch_on21/2, Switch_on20/2, Switch_on19/2, Switch_on18/2, Switch_on12/2, Switch_on10/2, Switch_on9/2, Switch_on8/2
  delayMatch/1 -> delayMatch141/1
  delayMatch1/1 -> delayMatch142/1
  Switch_on90/1 -> Subsystem/1(d_phase_voltage_per_switching_state), Delay135_enbsw/1
  Switch_on89/1 -> Subsystem/2(q_phase_voltage_per_switching_state), Delay134_enbsw/1
  Switch_on88/1 -> Subsystem/3(x_phase_voltage_per_switching_state), Delay133_enbsw/1
  Switch_on87/1 -> Subsystem/4(y_phase_voltage_per_switching_state), Delay132_enbsw/1
  Switch_on86/1 -> Subsystem/5(d_phase_voltage_per_switching_state1), Delay131_enbsw/1
  Switch_on85/1 -> Subsystem/6(q_phase_voltage_per_switching_state1), Delay130_enbsw/1
  Switch_on84/1 -> Subsystem/7(x_phase_voltage_per_switching_state1), Delay129_enbsw/1
  Switch_on83/1 -> Subsystem/8(y_phase_voltage_per_switching_state1), Delay128_enbsw/1
  Switch_on82/1 -> Subsystem/9(d_phase_voltage_per_switching_state2), Delay127_enbsw/1
  Switch_on81/1 -> Subsystem/10(q_phase_voltage_per_switching_state2), Delay126_enbsw/1
  Switch_on80/1 -> Subsystem/11(x_phase_voltage_per_switching_state2), Delay125_enbsw/1
  Switch_on79/1 -> Subsystem/12(y_phase_voltage_per_switching_state2), Delay124_enbsw/1
  Switch_on78/1 -> Subsystem/13(d_phase_voltage_per_switching_state3), Delay123_enbsw/1
  Switch_on77/1 -> Subsystem/14(q_phase_voltage_per_switching_state3), Delay122_enbsw/1
  Switch_on76/1 -> Subsystem/15(x_phase_voltage_per_switching_state3), Delay121_enbsw/1
  Switch_on75/1 -> Subsystem/16(y_phase_voltage_per_switching_state3), Delay120_enbsw/1
  Switch_on74/1 -> Subsystem/17(d_phase_voltage_per_switching_state4), Delay119_enbsw/1
  Switch_on73/1 -> Subsystem/18(q_phase_voltage_per_switching_state4), Delay118_enbsw/1
  Switch_on72/1 -> Subsystem/19(x_phase_voltage_per_switching_state4), Delay117_enbsw/1
  Switch_on71/1 -> Subsystem/20(y_phase_voltage_per_switching_state4), Delay116_enbsw/1
  Switch_on70/1 -> Subsystem/21(d_phase_voltage_per_switching_state5), Delay115_enbsw/1
  Switch_on69/1 -> Subsystem/22(q_phase_voltage_per_switching_state5), Delay114_enbsw/1
  Switch_on68/1 -> Subsystem/23(x_phase_voltage_per_switching_state5), Delay113_enbsw/1
  Switch_on67/1 -> Subsystem/24(y_phase_voltage_per_switching_state5), Delay112_enbsw/1
  Switch_on66/1 -> Subsystem/25(d_phase_voltage_per_switching_state6), Delay111_enbsw/1
  Switch_on65/1 -> Subsystem/26(q_phase_voltage_per_switching_state6), Delay110_enbsw/1
  Switch_on64/1 -> Subsystem/27(x_phase_voltage_per_switching_state6), Delay109_enbsw/1
  Switch_on63/1 -> Subsystem/28(y_phase_voltage_per_switching_state6), Delay108_enbsw/1
  Switch_on62/1 -> Subsystem/29(d_phase_voltage_per_switching_state7), Delay107_enbsw/1
  Switch_on61/1 -> Subsystem/30(q_phase_voltage_per_switching_state7), Delay106_enbsw/1
  Switch_on60/1 -> Subsystem/31(x_phase_voltage_per_switching_state7), Delay105_enbsw/1
  Switch_on59/1 -> Subsystem/32(y_phase_voltage_per_switching_state7), Delay104_enbsw/1
  Switch_on58/1 -> Subsystem/33(d_phase_voltage_per_switching_state8), Delay103_enbsw/1
  Switch_on57/1 -> Subsystem/34(q_phase_voltage_per_switching_state8), Delay102_enbsw/1
  Switch_on56/1 -> Subsystem/35(x_phase_voltage_per_switching_state8), Delay101_enbsw/1
  Switch_on55/1 -> Subsystem/36(y_phase_voltage_per_switching_state8), Delay100_enbsw/1
  Switch_on54/1 -> Subsystem/37(d_phase_voltage_per_switching_state9), Delay99_enbsw/1
  Switch_on53/1 -> Subsystem/38(q_phase_voltage_per_switching_state9), Delay98_enbsw/1
  Switch_on52/1 -> Subsystem/39(x_phase_voltage_per_switching_state9), Delay97_enbsw/1
  Switch_on51/1 -> Subsystem/40(y_phase_voltage_per_switching_state9), Delay96_enbsw/1
  Switch_on50/1 -> Subsystem/41(d_phase_voltage_per_switching_state10), Delay95_enbsw/1
  Switch_on49/1 -> Subsystem/42(q_phase_voltage_per_switching_state10), Delay94_enbsw/1
  Switch_on48/1 -> Subsystem/43(x_phase_voltage_per_switching_state10), Delay93_enbsw/1
  Switch_on47/1 -> Subsystem/44(y_phase_voltage_per_switching_state10), Delay92_enbsw/1
  Switch_on46/1 -> Subsystem/45(d_phase_voltage_per_switching_state11), Delay91_enbsw/1
  Switch_on45/1 -> Subsystem/46(q_phase_voltage_per_switching_state11), Delay90_enbsw/1
  Switch_on44/1 -> Subsystem/47(x_phase_voltage_per_switching_state11), Delay89_enbsw/1
  Switch_on43/1 -> Subsystem/48(y_phase_voltage_per_switching_state11), Delay88_enbsw/1
  Switch_on42/1 -> Subsystem/49(d_phase_voltage_per_switching_state12), Delay87_enbsw/1
  Switch_on41/1 -> Subsystem/50(q_phase_voltage_per_switching_state12), Delay86_enbsw/1
  Switch_on40/1 -> Subsystem/51(x_phase_voltage_per_switching_state12), Delay85_enbsw/1
  Switch_on39/1 -> Subsystem/52(y_phase_voltage_per_switching_state12), Delay84_enbsw/1
  Switch_on38/1 -> Subsystem/53(d_phase_voltage_per_switching_state13), Delay83_enbsw/1
  Switch_on37/1 -> Subsystem/54(q_phase_voltage_per_switching_state13), Delay82_enbsw/1
  Switch_on36/1 -> Subsystem/55(x_phase_voltage_per_switching_state13), Delay81_enbsw/1
  Switch_on35/1 -> Subsystem/56(y_phase_voltage_per_switching_state13), Delay80_enbsw/1
  Switch_on34/1 -> Subsystem/57(d_phase_voltage_per_switching_state14), Delay79_enbsw/1
  Switch_on33/1 -> Subsystem/58(q_phase_voltage_per_switching_state14), Delay78_enbsw/1
  Switch_on32/1 -> Subsystem/59(x_phase_voltage_per_switching_state14), Delay77_enbsw/1
  Switch_on31/1 -> Subsystem/60(y_phase_voltage_per_switching_state14), Delay76_enbsw/1
  Switch_on17/1 -> Subsystem/65(id_k_16), Delay16_enbsw/1
  Switch_on16/1 -> Subsystem/66(iq_k_16), Delay15_enbsw/1
  Switch_on15/1 -> Subsystem/67(ix_k_16), Delay14_enbsw/1
  Switch_on13/1 -> Subsystem/68(iy_k_16), Delay13_enbsw/1
  Switch_on11/1 -> Subsystem/70(omega_el15), Delay11_enbsw/1
  Switch_on7/1 -> Subsystem/74(d_phase_voltage_per_switching_state15), Delay7_enbsw/1
  Switch_on6/1 -> Subsystem/75(q_phase_voltage_per_switching_state15), Delay6_enbsw/1
  Switch_on5/1 -> Subsystem/76(x_phase_voltage_per_switching_state15), Delay5_enbsw/1
  Switch_on4/1 -> Subsystem/77(y_phase_voltage_per_switching_state15), Delay4_enbsw/1
  adder/1 -> switchEnable/3
  switchEnable/1 -> switchReset/3
  switchReset/1 -> HDL Counter/1
  Delay135_enbsw/1 -> Delay135/1
  Delay135/1 -> Switch_on90/3, Delay135_enbsw/3
  Delay134_enbsw/1 -> Delay134/1
  Delay134/1 -> Switch_on89/3, Delay134_enbsw/3
  Delay133_enbsw/1 -> Delay133/1
  Delay133/1 -> Switch_on88/3, Delay133_enbsw/3
  Delay132_enbsw/1 -> Delay132/1
  Delay132/1 -> Switch_on87/3, Delay132_enbsw/3
  Delay131_enbsw/1 -> Delay131/1
  Delay131/1 -> Switch_on86/3, Delay131_enbsw/3
  Delay130_enbsw/1 -> Delay130/1
  Delay130/1 -> Switch_on85/3, Delay130_enbsw/3
  Delay129_enbsw/1 -> Delay129/1
  Delay129/1 -> Switch_on84/3, Delay129_enbsw/3
  Delay128_enbsw/1 -> Delay128/1
  Delay128/1 -> Switch_on83/3, Delay128_enbsw/3
  Delay127_enbsw/1 -> Delay127/1
  Delay127/1 -> Switch_on82/3, Delay127_enbsw/3
  Delay126_enbsw/1 -> Delay126/1
  Delay126/1 -> Switch_on81/3, Delay126_enbsw/3
  Delay125_enbsw/1 -> Delay125/1
  Delay125/1 -> Switch_on80/3, Delay125_enbsw/3
  Delay124_enbsw/1 -> Delay124/1
  Delay124/1 -> Switch_on79/3, Delay124_enbsw/3
  Delay123_enbsw/1 -> Delay123/1
  Delay123/1 -> Switch_on78/3, Delay123_enbsw/3
  Delay122_enbsw/1 -> Delay122/1
  Delay122/1 -> Switch_on77/3, Delay122_enbsw/3
  Delay121_enbsw/1 -> Delay121/1
  Delay121/1 -> Switch_on76/3, Delay121_enbsw/3
  Delay120_enbsw/1 -> Delay120/1
  Delay120/1 -> Switch_on75/3, Delay120_enbsw/3
  Delay119_enbsw/1 -> Delay119/1
  Delay119/1 -> Switch_on74/3, Delay119_enbsw/3
  Delay118_enbsw/1 -> Delay118/1
  Delay118/1 -> Switch_on73/3, Delay118_enbsw/3
  Delay117_enbsw/1 -> Delay117/1
  Delay117/1 -> Switch_on72/3, Delay117_enbsw/3
  Delay116_enbsw/1 -> Delay116/1
  Delay116/1 -> Switch_on71/3, Delay116_enbsw/3
  Delay115_enbsw/1 -> Delay115/1
  Delay115/1 -> Switch_on70/3, Delay115_enbsw/3
  Delay114_enbsw/1 -> Delay114/1
  Delay114/1 -> Switch_on69/3, Delay114_enbsw/3
  Delay113_enbsw/1 -> Delay113/1
  Delay113/1 -> Switch_on68/3, Delay113_enbsw/3
  Delay112_enbsw/1 -> Delay112/1
  Delay112/1 -> Switch_on67/3, Delay112_enbsw/3
  Delay111_enbsw/1 -> Delay111/1
  Delay111/1 -> Switch_on66/3, Delay111_enbsw/3
  Delay110_enbsw/1 -> Delay110/1
  Delay110/1 -> Switch_on65/3, Delay110_enbsw/3
  Delay109_enbsw/1 -> Delay109/1
  Delay109/1 -> Switch_on64/3, Delay109_enbsw/3
  Delay108_enbsw/1 -> Delay108/1
  Delay108/1 -> Switch_on63/3, Delay108_enbsw/3
  Delay107_enbsw/1 -> Delay107/1
  Delay107/1 -> Switch_on62/3, Delay107_enbsw/3
  Delay106_enbsw/1 -> Delay106/1
  Delay106/1 -> Switch_on61/3, Delay106_enbsw/3
  Delay105_enbsw/1 -> Delay105/1
  Delay105/1 -> Switch_on60/3, Delay105_enbsw/3
  Delay104_enbsw/1 -> Delay104/1
  Delay104/1 -> Switch_on59/3, Delay104_enbsw/3
  Delay103_enbsw/1 -> Delay103/1
  Delay103/1 -> Switch_on58/3, Delay103_enbsw/3
  Delay102_enbsw/1 -> Delay102/1
  Delay102/1 -> Switch_on57/3, Delay102_enbsw/3
  Delay101_enbsw/1 -> Delay101/1
  Delay101/1 -> Switch_on56/3, Delay101_enbsw/3
  Delay100_enbsw/1 -> Delay100/1
  Delay100/1 -> Switch_on55/3, Delay100_enbsw/3
  Delay99_enbsw/1 -> Delay99/1
  Delay99/1 -> Switch_on54/3, Delay99_enbsw/3
  Delay98_enbsw/1 -> Delay98/1
  Delay98/1 -> Switch_on53/3, Delay98_enbsw/3
  Delay97_enbsw/1 -> Delay97/1
  Delay97/1 -> Switch_on52/3, Delay97_enbsw/3
  Delay96_enbsw/1 -> Delay96/1
  Delay96/1 -> Switch_on51/3, Delay96_enbsw/3
  Delay95_enbsw/1 -> Delay95/1
  Delay95/1 -> Switch_on50/3, Delay95_enbsw/3
  Delay94_enbsw/1 -> Delay94/1
  Delay94/1 -> Switch_on49/3, Delay94_enbsw/3
  Delay93_enbsw/1 -> Delay93/1
  Delay93/1 -> Switch_on48/3, Delay93_enbsw/3
  Delay92_enbsw/1 -> Delay92/1
  Delay92/1 -> Switch_on47/3, Delay92_enbsw/3
  Delay91_enbsw/1 -> Delay91/1
  Delay91/1 -> Switch_on46/3, Delay91_enbsw/3
  Delay90_enbsw/1 -> Delay90/1
  Delay90/1 -> Switch_on45/3, Delay90_enbsw/3
  Delay89_enbsw/1 -> Delay89/1
  Delay89/1 -> Switch_on44/3, Delay89_enbsw/3
  Delay88_enbsw/1 -> Delay88/1
  Delay88/1 -> Switch_on43/3, Delay88_enbsw/3
  Delay87_enbsw/1 -> Delay87/1
  Delay87/1 -> Switch_on42/3, Delay87_enbsw/3
  Delay86_enbsw/1 -> Delay86/1
  Delay86/1 -> Switch_on41/3, Delay86_enbsw/3
  Delay85_enbsw/1 -> Delay85/1
  Delay85/1 -> Switch_on40/3, Delay85_enbsw/3
  Delay84_enbsw/1 -> Delay84/1
  Delay84/1 -> Switch_on39/3, Delay84_enbsw/3
  Delay83_enbsw/1 -> Delay83/1
  Delay83/1 -> Switch_on38/3, Delay83_enbsw/3
  Delay82_enbsw/1 -> Delay82/1
  Delay82/1 -> Switch_on37/3, Delay82_enbsw/3
  Delay81_enbsw/1 -> Delay81/1
  Delay81/1 -> Switch_on36/3, Delay81_enbsw/3
  Delay80_enbsw/1 -> Delay80/1
  Delay80/1 -> Switch_on35/3, Delay80_enbsw/3
  Delay79_enbsw/1 -> Delay79/1
  Delay79/1 -> Switch_on34/3, Delay79_enbsw/3
  Delay78_enbsw/1 -> Delay78/1
  Delay78/1 -> Switch_on33/3, Delay78_enbsw/3
  Delay77_enbsw/1 -> Delay77/1
  Delay77/1 -> Switch_on32/3, Delay77_enbsw/3
  Delay76_enbsw/1 -> Delay76/1
  Delay76/1 -> Switch_on31/3, Delay76_enbsw/3
  Delay20/1 -> Switch_on21/3
  Delay19/1 -> Switch_on20/3
  Delay18/1 -> Switch_on19/3
  Delay17/1 -> Switch_on18/3
  Delay16_enbsw/1 -> Delay16/1
  Delay16/1 -> Switch_on17/3, Delay16_enbsw/3
  Delay15_enbsw/1 -> Delay15/1
  Delay15/1 -> Switch_on16/3, Delay15_enbsw/3
  Delay14_enbsw/1 -> Delay14/1
  Delay14/1 -> Switch_on15/3, Delay14_enbsw/3
  Delay13_enbsw/1 -> Delay13/1
  Delay13/1 -> Switch_on13/3, Delay13_enbsw/3
  Delay12/1 -> Switch_on12/3
  Delay11_enbsw/1 -> Delay11/1
  Delay11/1 -> Switch_on11/3, Delay11_enbsw/3
  Delay10/1 -> Switch_on10/3
  Delay9/1 -> Switch_on9/3
  Delay8/1 -> Switch_on8/3
  Delay7_enbsw/1 -> Delay7/1
  Delay7/1 -> Switch_on7/3, Delay7_enbsw/3
  Delay6_enbsw/1 -> Delay6/1
  Delay6/1 -> Switch_on6/3, Delay6_enbsw/3
  Delay5_enbsw/1 -> Delay5/1
  Delay5/1 -> Switch_on5/3, Delay5_enbsw/3
  Delay4_enbsw/1 -> Delay4/1
  Delay4/1 -> Switch_on4/3, Delay4_enbsw/3

== system gm_parallel_prediction_and_cost_function_6phase/Prediction_and_cost_function/Compare To Constant ==
  u : Inport  OutDataTypeStr=fixdt(1,32,0,'DataTypeOverride', 'Off')  SampleTime=1e-08
  Compare : RelationalOperator  Operator=<=  OutDataTypeStr=boolean
  Constant : Constant  DisableCoverage=on  Value=const  OutDataTypeStr=Inherit: Inherit via back propagation  SampleTime=-1
  y : Outport  SampleTime=1e-08
  wires:
  Compare/1 -> y/1
  Constant/1 -> Compare/2
  u/1 -> Compare/1

== system gm_parallel_prediction_and_cost_function_6phase/Prediction_and_cost_function/Data Type Conversion1 ==
  In1 : Inport
  Data Type Conversion1 : DataTypeConversion  OutDataTypeStr=single  RndMeth=Nearest  SampleTime=1e-08  SaturateOnIntegerOverflow=off
  Data Type Conversion1_pd1 : Delay  DelayLength=6
  Out1 : Outport
  wires:
  In1/1 -> Data Type Conversion1/1
  Data Type Conversion1/1 -> Data Type Conversion1_pd1/1
  Data Type Conversion1_pd1/1 -> Out1/1

== system gm_parallel_prediction_and_cost_function_6phase/Prediction_and_cost_function/Data Type Conversion10 ==
  In1 : Inport
  Data Type Conversion10 : DataTypeConversion  OutDataTypeStr=single  RndMeth=Nearest  SampleTime=1e-08  SaturateOnIntegerOverflow=off
  Data Type Conversion10_pd1 : Delay  DelayLength=6
  Out1 : Outport
  wires:
  In1/1 -> Data Type Conversion10/1
  Data Type Conversion10/1 -> Data Type Conversion10_pd1/1
  Data Type Conversion10_pd1/1 -> Out1/1

== system gm_parallel_prediction_and_cost_function_6phase/Prediction_and_cost_function/Data Type Conversion18 ==
  In1 : Inport
  Data Type Conversion18 : DataTypeConversion  OutDataTypeStr=fixdt(1, 18, 11)  RndMeth=Nearest  SampleTime=1e-08  SaturateOnIntegerOverflow=off
  Data Type Conversion18_pd1 : Delay  DelayLength=6
  Out1 : Outport
  wires:
  In1/1 -> Data Type Conversion18/1
  Data Type Conversion18/1 -> Data Type Conversion18_pd1/1
  Data Type Conversion18_pd1/1 -> Out1/1

== system gm_parallel_prediction_and_cost_function_6phase/Prediction_and_cost_function/Data Type Conversion4 ==
  In1 : Inport
  Data Type Conversion4 : DataTypeConversion  OutDataTypeStr=single  RndMeth=Nearest  SampleTime=1e-08  SaturateOnIntegerOverflow=off
  Data Type Conversion4_pd1 : Delay  DelayLength=6
  Out1 : Outport
  wires:
  In1/1 -> Data Type Conversion4/1
  Data Type Conversion4/1 -> Data Type Conversion4_pd1/1
  Data Type Conversion4_pd1/1 -> Out1/1

== system gm_parallel_prediction_and_cost_function_6phase/Prediction_and_cost_function/Data Type Conversion7 ==
  In1 : Inport
  Data Type Conversion7 : DataTypeConversion  OutDataTypeStr=single  RndMeth=Nearest  SampleTime=1e-08  SaturateOnIntegerOverflow=off
  Data Type Conversion7_pd1 : Delay  DelayLength=6
  Out1 : Outport
  wires:
  In1/1 -> Data Type Conversion7/1
  Data Type Conversion7/1 -> Data Type Conversion7_pd1/1
  Data Type Conversion7_pd1/1 -> Out1/1

== system gm_parallel_prediction_and_cost_function_6phase/Prediction_and_cost_function/Data Type Conversion8 ==
  In1 : Inport
  Data Type Conversion8 : DataTypeConversion  OutDataTypeStr=single  RndMeth=Nearest  SampleTime=1e-08  SaturateOnIntegerOverflow=off
  Data Type Conversion8_pd1 : Delay  DelayLength=6
  Out1 : Outport
  wires:
  In1/1 -> Data Type Conversion8/1
  Data Type Conversion8/1 -> Data Type Conversion8_pd1/1
  Data Type Conversion8_pd1/1 -> Out1/1

== system gm_parallel_prediction_and_cost_function_6phase/Prediction_and_cost_function/Data Type Conversion9 ==
  In1 : Inport
  Data Type Conversion9 : DataTypeConversion  OutDataTypeStr=single  RndMeth=Nearest  SampleTime=1e-08  SaturateOnIntegerOverflow=off
  Data Type Conversion9_pd1 : Delay  DelayLength=6
  Out1 : Outport
  wires:
  In1/1 -> Data Type Conversion9/1
  Data Type Conversion9/1 -> Data Type Conversion9_pd1/1
  Data Type Conversion9_pd1/1 -> Out1/1
